simulink model "kapitsa_pendulum"  (R2021b)
settings: Solver=VariableStepAuto  StartTime=0.0  StopTime=30  MaxStep=0.05  RelTol=1e-3
undefined symbols (not defined in the file): b, l, phi, w
libraries: simulink_extras x1
settings Model: Creator=user  LastModifiedBy=user
settings DataIOCC: ReturnWorkspaceOutputs=off

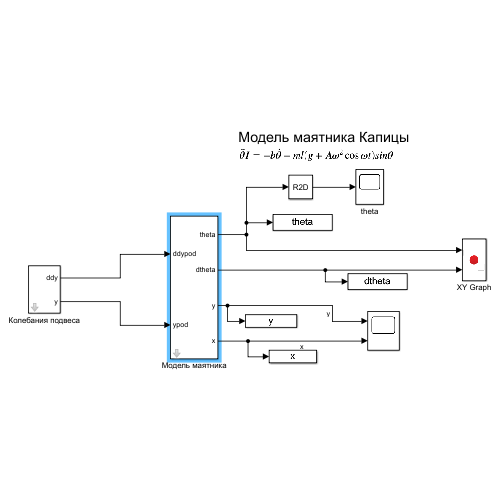
[thumbnail: Simulink's stored preview of the top-level diagram]
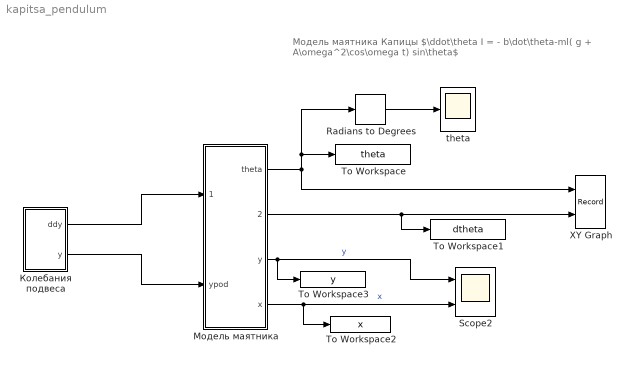
== system kapitsa_pendulum ==
  note: Модель маятника Капицы
      | $\ddot\theta I = - b\dot\theta-ml( g + A\omega^2\cos\omega t) sin\theta$
  Radians to Degrees : simulink_extras/Transformations/Radians to Degrees
  Scope2 : Scope  NumInputPorts=2
  To Workspace : ToWorkspace  VariableName=theta  SampleTime=-1
      settings: Save2DSignal=2-D array (concatenate along first dimension)
  To Workspace1 : ToWorkspace  VariableName=dtheta  SampleTime=-1
      settings: Save2DSignal=2-D array (concatenate along first dimension)
  To Workspace2 : ToWorkspace  VariableName=x  SampleTime=-1
      settings: Save2DSignal=2-D array (concatenate along first dimension)
  To Workspace3 : ToWorkspace  VariableName=y  SampleTime=-1
      settings: Save2DSignal=2-D array (concatenate along first dimension)
  XY Graph : Record  FileSettingsInternal="{\"entries\":[{\"content\":{\"excelSettings\":{\"content\":{},\"type\":\"Streamout.ExcelSettings\"}},\"type\":\"Streamout.FileSettingStorage\",\"uuid\":\"d8596cab-30da-49a5-bac1-1ead71a79572\"}],\"packageUris\":[\"http://schema.mathworks.com/mf0/streamout_blocks/R2020a\"],\"version\":\"1.0\"}"  Layout=[1 1]  SignalsInternal="{\"entries\":[{\"content\":{\"signals\":[{\"content\":{\"blockPath\":[\"kapitsa_pendulum/XY Graph\"],\"channel\":[],\"dimensions\":[1],\"domain\":\"kapitsa_pendulum/XY Graph\",\"lineColor\":\"#a2142f\",\"plots\":[1],\"port\":1,\"sid\":[\"\"],\"signalID\":2918,\"signalName\":\"Модель маятника:1\"},\"type\":\"RecordBlkView.Signal\",\"uuid\":\"0486ef19-4123-4802-91da-7f0958843597\"},{\"content\":{\"blockPath\":[\"kapitsa_pendulum/XY Graph\"],\"channel\":[],\"dimensions\":[1],\"domain\":\"kapitsa_pendulum/XY Graph\",\"lineColor\":\"#139fff\",\"plots\":[1],\"port\":2,\"sid\":[\"\"],\"signalID\":2922,\"signalName\":\"Модель маятника:2\"},\"type\":\"RecordBlkView.Signal\",\"uuid\":\"4c794a1e-d859-44f5-b011-bed80ad5a9b8\"}]},\"type\":\"RecordBlkView.InputSignals\",\"uuid\":\"3d8bb8d7-54bb-46dc-98e9-398a5f531cfc\"}],\"packageUris\":[\"http://schema.mathworks.com/mf0/streamout_blocks/R2020a\"],\"version\":\"1.0\"}"  VisualizationBindings="{\"xyplotplugin\":{\"info\":[{\"series\":[{\"bindingParametersList\":[{\"parameter\":\"X-Axis\",\"signalID\":2918,\"signalName\":\"РњРѕРґРµР»СЊ РјР°СЏС‚РЅРёРєР°:1\"},{\"parameter\":\"Y-Axis\",\"signalID\":2922,\"signalName\":\"РњРѕРґРµР»СЊ РјР°СЏС‚РЅРёРєР°:2\"}],\"seriesID\":57799}],\"subplotID\":1}]}}"  CompatibilityTag=XY
  theta : Scope
  Колебания подвеса : Subsystem  mask{A=l, w=w}
      mask prompts: A "амплитуда"; w "угловая скорость"
  Модель маятника : Subsystem  mask{m=1, l=10, g=9.8, startDegree=phi, b=b}
      mask prompts: m "масса"; l "длина подвеса"; g "ускорение свободного падения"; startDegree "стартовый угол"; b "диссипативный член"
      mask init:
      | I = m * l^2
  wires:
  Модель маятника/4(x) -> To Workspace2/1, Scope2/2  "x"
  Модель маятника/3(y) -> Scope2/1, To Workspace3/1  "y"
  Модель маятника/1(theta) -> Radians to Degrees/1, To Workspace/1, XY Graph/1
  Модель маятника/2(dtheta) -> To Workspace1/1, XY Graph/2
  Radians to Degrees/1 -> theta/1
  Колебания подвеса/1(ddy) -> Модель маятника/1(ddypod)
  Колебания подвеса/2(y) -> Модель маятника/2(ypod)

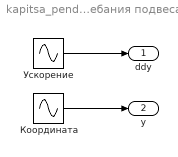
== system kapitsa_pendulum/Колебания подвеса ==
  Координата : Sin  Amplitude=A  Frequency=w * (2 * pi)  Phase=pi/2  SampleTime=0
  Ускорение : Sin  Amplitude=-A * (w * (2* pi))^2  Frequency=w * (2* pi)  Phase=pi/2  SampleTime=0
  ddy : Outport
  y : Outport  Port=2
  wires:
  Ускорение/1 -> ddy/1
  Координата/1 -> y/1

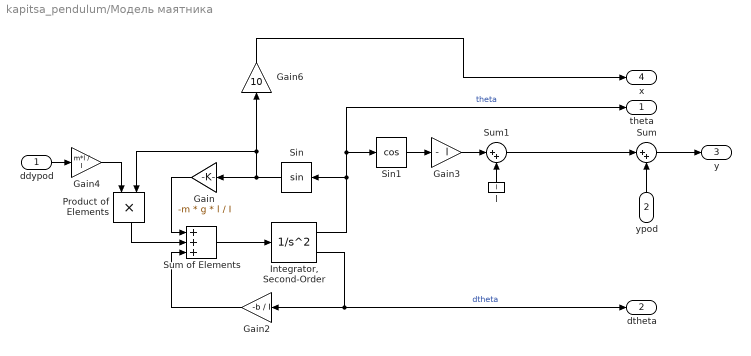
== system kapitsa_pendulum/Модель маятника ==
  ddypod : Inport
  ypod : Inport  Port=2
  Gain : Gain  Gain=-m * g * l / I
  Gain2 : Gain  Gain=-b / I
  Gain3 : Gain  Gain="-  l"
  Gain4 : Gain  Gain=m*l / I
  Gain6 : Gain  Gain=10
  "Integrator, Second-Order" : SecondOrderIntegrator  ICX=deg2rad(startDegree)
  Product of Elements : Product  Inputs=**
  Sin : Trigonometry
  Sin1 : Trigonometry  Operator=cos
  Sum : Sum  Inputs=|++
  Sum of Elements : Sum  Inputs=+++
  Sum1 : Sum  Inputs=|++
  l : Constant  Value=l
  theta : Outport
  dtheta : Outport  Port=2
  y : Outport  Port=3
  x : Outport  Port=4
  wires:
  Sin/1 -> Gain/1, Gain6/1, Product of Elements/2
  "Integrator, Second-Order"/1 -> Sin1/1, theta/1, Sin/1  "theta"
  "Integrator, Second-Order"/2 -> Gain2/1, dtheta/1  "dtheta"
  Gain/1 -> Sum of Elements/1
  Gain2/1 -> Sum of Elements/3
  Sin1/1 -> Gain3/1
  l/1 -> Sum1/2
  Gain3/1 -> Sum1/1
  Gain6/1 -> x/1
  ddypod/1 -> Gain4/1
  Gain4/1 -> Product of Elements/1
  Product of Elements/1 -> Sum of Elements/2
  Sum of Elements/1 -> "Integrator, Second-Order"/1
  Sum1/1 -> Sum/1
  Sum/1 -> y/1
  ypod/1 -> Sum/2
